simulink model "step9_power_4"  (R2025a)
settings: Solver=ode45  StartTime=0.0  StopTime=20  MaxStep=0.01  RelTol=1e-3
undefined symbols (not defined in the file or in its folder): A, B, F, K, R
libraries: SignalEditorBlockLib x1
settings Model: Creator=O M E N  LastModifiedBy=O M E N

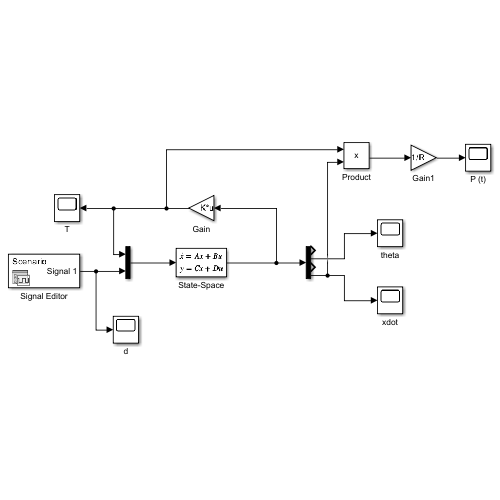
[thumbnail: Simulink's stored preview of the top-level diagram]
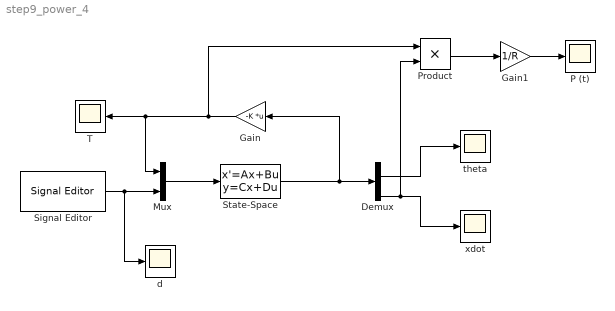
== system step9_power_4 ==
  Demux : Demux
  Gain : Gain  Gain=-K  Multiplication=Matrix(K*u)
  Gain1 : Gain  Gain=1/R
  Mux : Mux  Inputs=2
  P (t) : Scope
      settings: Title=Mechanical power P(t)  ActiveDisplayYMinimum=-9.25899114539923  ActiveDisplayYMaximum=32.994756051505092  YLabel="P  (W)"  DataLoggingVariableName=ScopeData4
  Product : Product
  Signal Editor : SignalEditorBlockLib/Signal Editor  FileName=d_trapezoid.mat  ActiveScenario=Scenario  ActiveSignal=Signal 1  IsBus=off  OutputBusObjectStr=Bus: BusObject  SampleTime=0  ZeroCross=off  OutputAfterFinalValue=Setting to zero  Unit=inherit  PreserveSignalName=on  ApplySigPropsToAllScenarios=on  ApplySigPropsToAllSignals=off  SignalPropertySource=Dialog parameters
  State-Space : StateSpace  A=A  B=[B F]  C=eye(4)  D=zeros(4,2)  InitialCondition=[0; 0; 0; 0]
  T : Scope
      settings: Title=Control torque T(t)  ActiveDisplayYMinimum=-3.0690975343920019  ActiveDisplayYMaximum=11.898097533737634  YLabel="T  (N·m)"  DataLoggingVariableName=ScopeData2
  d : Scope
      settings: Title=Disturbance d(t)  ActiveDisplayYMinimum=-0.0012499999999999998  ActiveDisplayYMaximum=0.01125  YLabel="d  (m)"  DataLoggingVariableName=ScopeData3
  theta : Scope
      settings: Title=Tilt angle θ(t)  ActiveDisplayYMinimum=-0.0014361778362387047  ActiveDisplayYMaximum=0.0014361778372283518  YLabel="θ  (rad)"
  xdot : Scope
      settings: Title=Vehicle speed ẋ(t)  ActiveDisplayYMinimum=-0.14676890030256073  ActiveDisplayYMaximum=1.3209201027230468  YLabel="ẋ  (m/s)"
  wires:
  Mux/1 -> State-Space/1
  State-Space/1 -> Gain/1, Demux/1
  Demux/2 -> theta/1
  Demux/4 -> Product/2, xdot/1
  Gain/1 -> Product/1, T/1, Mux/1
  Signal Editor/1 -> d/1, Mux/2
  Product/1 -> Gain1/1
  Gain1/1 -> P (t)/1
